simulink model "wecSim"  (R2016b)
settings: Solver=ode3  StartTime=0.0  StopTime=mdl.tEnd  FixedStep=mdl.tStep  RelTol=1e-3
undefined symbols (not defined in the file): ics, magnitude, nextDelatchTime, pto
settings Model: Creator=ggparker  LastModifiedBy=s1343354
settings DataIOCC: SaveFinalState=on  SaveCompleteFinalSimState=on  SaveOutput=off  SaveTime=off

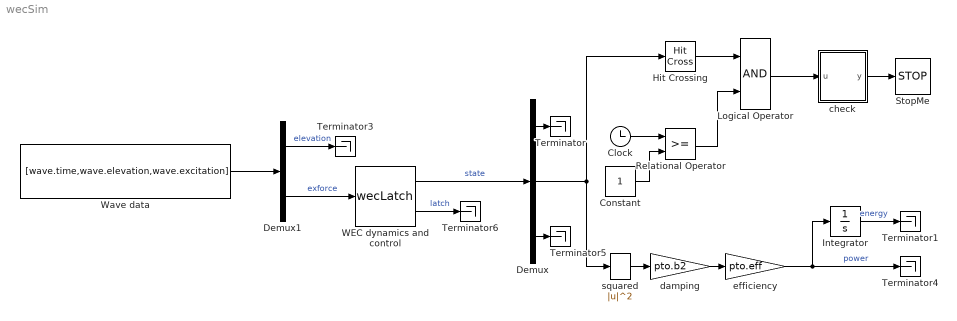
== system wecSim ==
  Clock : Clock
  Constant : Constant
  Demux : Demux  Outputs=[3; 1; 4]
  Demux1 : Demux  Outputs=[1; 1]
  Hit Crossing : HitCross
  Integrator : Integrator
  Logical Operator : Logic  AllPortsSameDT=off  OutDataTypeStr=boolean
  Relational Operator : RelationalOperator  OutDataTypeStr=boolean  RndMeth=Simplest
  StopMe : Stop
  Terminator{,1,3..6} (6 alike) : Terminator
  WEC dynamics and control : S-Function  FunctionName=wecLatch  Parameters=nextDelatchTime,ss.A',ss.B',ics  SFunctionDeploymentMode=off  EnableBusSupport=off
  Wave data : FromWorkspace  VariableName=[wave.time,wave.elevation,wave.excitation]  SampleTime=0
  check : MATLAB Function  TreatAsAtomicUnit=on
  damping : Gain  Gain=pto.b2
  efficiency : Gain  Gain=pto.eff
  squared : Math  Operator=magnitude^2  SaturateOnIntegerOverflow=on
  wires:
  efficiency/1 -> Terminator4/1, Integrator/1  "power"
  WEC dynamics and control/1 -> Demux/1  "state"
  Wave data/1 -> Demux1/1
  Demux1/1 -> Terminator3/1  "elevation"
  Integrator/1 -> Terminator1/1  "energy"
  Demux1/2 -> WEC dynamics and control/1  "exforce"
  damping/1 -> efficiency/1
  Demux/2 -> squared/1, Hit Crossing/1
  Clock/1 -> Relational Operator/1
  Constant/1 -> Relational Operator/2
  Hit Crossing/1 -> Logical Operator/1
  Relational Operator/1 -> Logical Operator/2
  Logical Operator/1 -> check/1(u)
  check/1(y) -> StopMe/1
  Demux/1 -> Terminator/1
  Demux/3 -> Terminator5/1
  squared/1 -> damping/1
  WEC dynamics and control/2 -> Terminator6/1  "latch"

== matlab function wecSim/check ==
  data: u input; y output; c parameter
function y = fcn(u,c)
% fcn.m      E.Anderlini@ed.ac.uk     07/03/2017
%%%%%%%%%%%%%%%%%%%%%%%%%%%%%%%%%%%%%%%%%%%%%%%%%%%%%%%%%%%%%%%%%%%%%%%%%%%
% This function sets the exit flag for the simulation.
%%%%%%%%%%%%%%%%%%%%%%%%%%%%%%%%%%%%%%%%%%%%%%%%%%%%%%%%%%%%%%%%%%%%%%%%%%%

%% Define and initialize a counter:
persistent counter;
if isempty(counter)
    counter = 0;
end

%% Set the exit flag:
% Initialize the exit flag to false:
y = false;
% Update the counter if v2 has a zero crossing:
if u
    counter = counter + 1;
end
% Stop the simulation only after a full wave cycle or until the end:
if counter>1 && c<1
    % Set the exit flag to true:
    y = true;
    % Reset the counter:
    counter = 0;
end

end
